simulink model "Pendulum"  (R2017b)
settings: Solver=VariableStepAuto  StartTime=0.0  StopTime=10.0  MaxStep=0.001  RelTol=1e-3
settings Model: Creator=guoro  LastModifiedBy=guoro

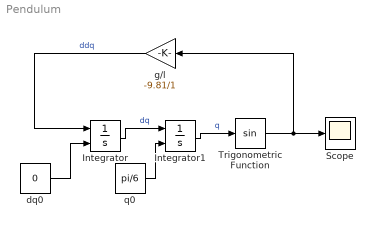
== system Pendulum ==
  Integrator : Integrator  InitialConditionSource=external
  Integrator1 : Integrator  InitialConditionSource=external
  Scope : Scope
  Trigonometric Function : Trigonometry
  dq0 : Constant  Value=0
  g/l : Gain  Gain=-9.81/1
  q0 : Constant  Value=pi/6
  wires:
  Integrator/1 -> Integrator1/1  "dq"
  g/l/1 -> Integrator/1  "ddq"
  Integrator1/1 -> Trigonometric Function/1  "q"
  Trigonometric Function/1 -> Scope/1, g/l/1
  dq0/1 -> Integrator/2
  q0/1 -> Integrator1/2
